simulink library "vlbi_lib"  (Simulink 7.3)
settings: Solver=ode45  SolverMode=SingleTasking  StartTime=0.0  StopTime=10.0  RelTol=1e-3
libraries: xbsIndex_r4 x437, xbsReplacements_r4 x26, simulink x3, xps_library x2
(part 2 of 2)

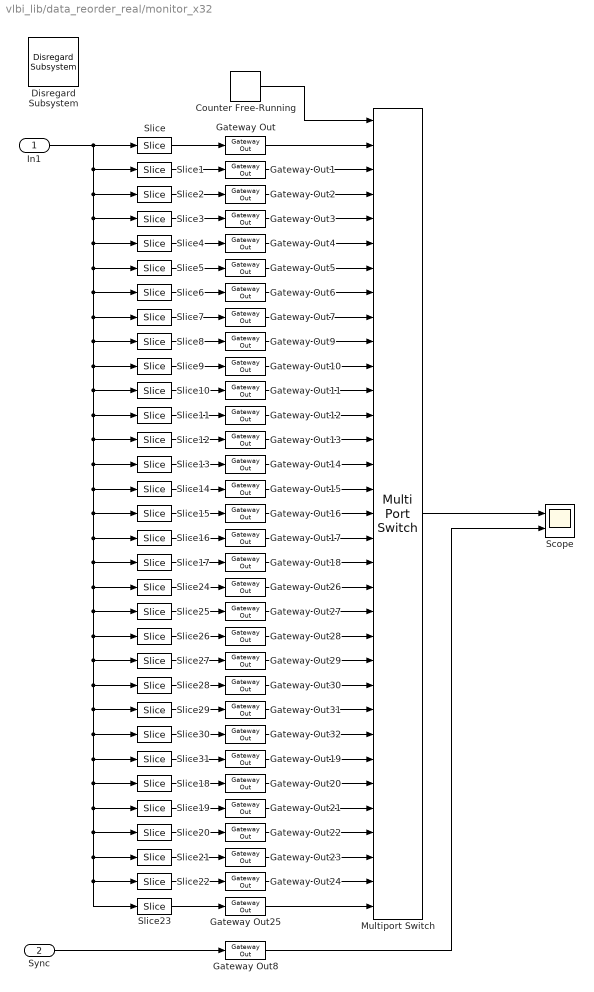
== system vlbi_lib/data_reorder_real/monitor_x32 ==
  In1 : Inport  OutDataType=sfix(16)  OutScaling=2^0
  Sync : Inport  Port=2  OutDataType=sfix(16)  OutScaling=2^0
  Counter Free-Running : simulink/Sources/Counter Free-Running  SystemSampleTime=-1  NumBits=5  tsamp=1/32
  Disregard Subsystem : xbsIndex_r4/Disregard Subsystem  Tag=discardX  block_type=disregard
      settings: block_version=11.3
  Gateway Out{,1..32} (33 alike) : xbsIndex_r4/Gateway Out  hdl_port=off  timing_constraint=None  locs_specified=off  LOCs={}  block_type=gatewayout
      settings: infoedit="Gateway out block.  Converts Xilinx fixed point inputs into ouputs of type Simulink integer, double, or fixed point.<br><br>Hardware notes:  In hardware these blocks become top level output ports or are discarded, depending on how they are configured."  xl_area=[0, 0, 0, 0, 0, 0, 0]  block_version=11.3
  Multiport Switch : MultiPortSwitch  Inputs=32  zeroidx=on  SampleTime=1/32
  Scope : Scope  NumInputPorts=2
      settings: YMin=-5~-5  YMax=5~5
  Slice : xbsIndex_r4/Slice  nbits=sample_width  boolean_output=off  mode=Lower Bit Location + Width  bit1=sample_width*0  base1=MSB of Input  bit0=sample_width*7  base0=LSB of Input  dbl_ovrd=off  block_type=slice
      settings: block_version=11.3
  Slice1 : xbsIndex_r4/Slice  nbits=sample_width  boolean_output=off  mode=Lower Bit Location + Width  bit1=-2*sample_width  base1=MSB of Input  bit0=sample_width*6  base0=LSB of Input  dbl_ovrd=off  block_type=slice
      settings: block_version=11.3
  Slice10 : xbsIndex_r4/Slice  nbits=sample_width  boolean_output=off  mode=Lower Bit Location + Width  bit1=sample_width*21  base1=MSB of Input  bit0=sample_width*21  base0=LSB of Input  dbl_ovrd=off  block_type=slice
      settings: block_version=11.3
  Slice11 : xbsIndex_r4/Slice  nbits=sample_width  boolean_output=off  mode=Lower Bit Location + Width  bit1=-22*sample_width  base1=MSB of Input  bit0=sample_width*20  base0=LSB of Input  dbl_ovrd=off  block_type=slice
      settings: block_version=11.3
  Slice12 : xbsIndex_r4/Slice  nbits=sample_width  boolean_output=off  mode=Lower Bit Location + Width  bit1=-24*sample_width  base1=MSB of Input  bit0=sample_width*31  base0=LSB of Input  dbl_ovrd=off  block_type=slice
      settings: block_version=11.3
  Slice13 : xbsIndex_r4/Slice  nbits=sample_width  boolean_output=off  mode=Lower Bit Location + Width  bit1=-26*sample_width  base1=MSB of Input  bit0=sample_width*30  base0=LSB of Input  dbl_ovrd=off  block_type=slice
      settings: block_version=11.3
  Slice14 : xbsIndex_r4/Slice  nbits=sample_width  boolean_output=off  mode=Lower Bit Location + Width  bit1=-28*sample_width  base1=MSB of Input  bit0=sample_width*29  base0=LSB of Input  dbl_ovrd=off  block_type=slice
      settings: block_version=11.3
  Slice15 : xbsIndex_r4/Slice  nbits=sample_width  boolean_output=off  mode=Lower Bit Location + Width  bit1=-30*sample_width  base1=MSB of Input  bit0=sample_width*28  base0=LSB of Input  dbl_ovrd=off  block_type=slice
      settings: block_version=11.3
  Slice16 : xbsIndex_r4/Slice  nbits=sample_width  boolean_output=off  mode=Lower Bit Location + Width  bit1=-1*sample_width  base1=MSB of Input  bit0=sample_width*3  base0=LSB of Input  dbl_ovrd=off  block_type=slice
      settings: block_version=11.3
  Slice17 : xbsIndex_r4/Slice  nbits=sample_width  boolean_output=off  mode=Lower Bit Location + Width  bit1=-3*sample_width  base1=MSB of Input  bit0=sample_width*2  base0=LSB of Input  dbl_ovrd=off  block_type=slice
      settings: block_version=11.3
  Slice18 : xbsIndex_r4/Slice  nbits=sample_width  boolean_output=off  mode=Lower Bit Location + Width  bit1=-21*sample_width  base1=MSB of Input  bit0=sample_width*17  base0=LSB of Input  dbl_ovrd=off  block_type=slice
      settings: block_version=11.3
  Slice19 : xbsIndex_r4/Slice  nbits=sample_width  boolean_output=off  mode=Lower Bit Location + Width  bit1=-23*sample_width  base1=MSB of Input  bit0=sample_width*16  base0=LSB of Input  dbl_ovrd=off  block_type=slice
      settings: block_version=11.3
  Slice2 : xbsIndex_r4/Slice  nbits=sample_width  boolean_output=off  mode=Lower Bit Location + Width  bit1=-4*sample_width  base1=MSB of Input  bit0=sample_width*5  base0=LSB of Input  dbl_ovrd=off  block_type=slice
      settings: block_version=11.3
  Slice20 : xbsIndex_r4/Slice  nbits=sample_width  boolean_output=off  mode=Lower Bit Location + Width  bit1=-25*sample_width  base1=MSB of Input  bit0=sample_width*27  base0=LSB of Input  dbl_ovrd=off  block_type=slice
      settings: block_version=11.3
  Slice21 : xbsIndex_r4/Slice  nbits=sample_width  boolean_output=off  mode=Lower Bit Location + Width  bit1=-27*sample_width  base1=MSB of Input  bit0=sample_width*26  base0=LSB of Input  dbl_ovrd=off  block_type=slice
      settings: block_version=11.3
  Slice22 : xbsIndex_r4/Slice  nbits=sample_width  boolean_output=off  mode=Lower Bit Location + Width  bit1=-29*sample_width  base1=MSB of Input  bit0=sample_width*25  base0=LSB of Input  dbl_ovrd=off  block_type=slice
      settings: block_version=11.3
  Slice23 : xbsIndex_r4/Slice  nbits=sample_width  boolean_output=off  mode=Lower Bit Location + Width  bit1=-31*sample_width  base1=MSB of Input  bit0=sample_width*24  base0=LSB of Input  dbl_ovrd=off  block_type=slice
      settings: block_version=11.3
  Slice24 : xbsIndex_r4/Slice  nbits=sample_width  boolean_output=off  mode=Lower Bit Location + Width  bit1=-5*sample_width  base1=MSB of Input  bit0=sample_width*1  base0=LSB of Input  dbl_ovrd=off  block_type=slice
      settings: block_version=11.3
  Slice25 : xbsIndex_r4/Slice  nbits=sample_width  boolean_output=off  mode=Lower Bit Location + Width  bit1=-7*sample_width  base1=MSB of Input  bit0=sample_width*0  base0=LSB of Input  dbl_ovrd=off  block_type=slice
      settings: block_version=11.3
  Slice26 : xbsIndex_r4/Slice  nbits=sample_width  boolean_output=off  mode=Lower Bit Location + Width  bit1=-9*sample_width  base1=MSB of Input  bit0=sample_width*11  base0=LSB of Input  dbl_ovrd=off  block_type=slice
      settings: block_version=11.3
  Slice27 : xbsIndex_r4/Slice  nbits=sample_width  boolean_output=off  mode=Lower Bit Location + Width  bit1=-11*sample_width  base1=MSB of Input  bit0=sample_width*10  base0=LSB of Input  dbl_ovrd=off  block_type=slice
      settings: block_version=11.3
  Slice28 : xbsIndex_r4/Slice  nbits=sample_width  boolean_output=off  mode=Lower Bit Location + Width  bit1=-13*sample_width  base1=MSB of Input  bit0=sample_width*9  base0=LSB of Input  dbl_ovrd=off  block_type=slice
      settings: block_version=11.3
  Slice29 : xbsIndex_r4/Slice  nbits=sample_width  boolean_output=off  mode=Lower Bit Location + Width  bit1=-15*sample_width  base1=MSB of Input  bit0=sample_width*8  base0=LSB of Input  dbl_ovrd=off  block_type=slice
      settings: block_version=11.3
  Slice3 : xbsIndex_r4/Slice  nbits=sample_width  boolean_output=off  mode=Lower Bit Location + Width  bit1=-6*sample_width  base1=MSB of Input  bit0=sample_width*4  base0=LSB of Input  dbl_ovrd=off  block_type=slice
      settings: block_version=11.3
  Slice30 : xbsIndex_r4/Slice  nbits=sample_width  boolean_output=off  mode=Lower Bit Location + Width  bit1=-17*sample_width  base1=MSB of Input  bit0=sample_width*19  base0=LSB of Input  dbl_ovrd=off  block_type=slice
      settings: block_version=11.3
  Slice31 : xbsIndex_r4/Slice  nbits=sample_width  boolean_output=off  mode=Lower Bit Location + Width  bit1=sample_width*18  base1=MSB of Input  bit0=sample_width*18  base0=LSB of Input  dbl_ovrd=off  block_type=slice
      settings: block_version=11.3
  Slice4 : xbsIndex_r4/Slice  nbits=sample_width  boolean_output=off  mode=Lower Bit Location + Width  bit1=-8*sample_width  base1=MSB of Input  bit0=sample_width*15  base0=LSB of Input  dbl_ovrd=off  block_type=slice
      settings: block_version=11.3
  Slice5 : xbsIndex_r4/Slice  nbits=sample_width  boolean_output=off  mode=Lower Bit Location + Width  bit1=-10*sample_width  base1=MSB of Input  bit0=sample_width*14  base0=LSB of Input  dbl_ovrd=off  block_type=slice
      settings: block_version=11.3
  Slice6 : xbsIndex_r4/Slice  nbits=sample_width  boolean_output=off  mode=Lower Bit Location + Width  bit1=-12*sample_width  base1=MSB of Input  bit0=sample_width*13  base0=LSB of Input  dbl_ovrd=off  block_type=slice
      settings: block_version=11.3
  Slice7 : xbsIndex_r4/Slice  nbits=sample_width  boolean_output=off  mode=Lower Bit Location + Width  bit1=-14*sample_width  base1=MSB of Input  bit0=sample_width*12  base0=LSB of Input  dbl_ovrd=off  block_type=slice
      settings: block_version=11.3
  Slice8 : xbsIndex_r4/Slice  nbits=sample_width  boolean_output=off  mode=Lower Bit Location + Width  bit1=-16*sample_width  base1=MSB of Input  bit0=sample_width*23  base0=LSB of Input  dbl_ovrd=off  block_type=slice
      settings: block_version=11.3
  Slice9 : xbsIndex_r4/Slice  nbits=sample_width  boolean_output=off  mode=Lower Bit Location + Width  bit1=-18*sample_width  base1=MSB of Input  bit0=sample_width*22  base0=LSB of Input  dbl_ovrd=off  block_type=slice
      settings: block_version=11.3
  wires:
  Gateway Out8/1 -> Scope/2
  Sync/1 -> Gateway Out8/1
  Multiport Switch/1 -> Scope/1
  Counter Free-Running/1 -> Multiport Switch/1
  Slice7/1 -> Gateway Out7/1
  Slice6/1 -> Gateway Out6/1
  Slice5/1 -> Gateway Out5/1
  Slice4/1 -> Gateway Out4/1
  Slice3/1 -> Gateway Out3/1
  Slice2/1 -> Gateway Out2/1
  Slice1/1 -> Gateway Out1/1
  Slice/1 -> Gateway Out/1
  In1/1 -> Slice6/1, Slice7/1, Slice14/1, Slice15/1, Slice16/1, Slice17/1, Slice24/1, Slice25/1, Slice26/1, Slice27/1, Slice30/1, Slice31/1, Slice18/1, Slice19/1, Slice20/1, Slice21/1, Slice22/1, Slice23/1, Slice29/1, Slice28/1, Slice13/1, Slice12/1, Slice11/1, Slice10/1, Slice9/1, Slice8/1, Slice5/1, Slice4/1, Slice3/1, Slice2/1, Slice1/1, Slice/1
  Slice15/1 -> Gateway Out16/1
  Slice14/1 -> Gateway Out15/1
  Slice13/1 -> Gateway Out14/1
  Slice12/1 -> Gateway Out13/1
  Slice11/1 -> Gateway Out12/1
  Slice10/1 -> Gateway Out11/1
  Slice9/1 -> Gateway Out10/1
  Slice8/1 -> Gateway Out9/1
  Slice29/1 -> Gateway Out31/1
  Slice28/1 -> Gateway Out30/1
  Slice27/1 -> Gateway Out29/1
  Slice26/1 -> Gateway Out28/1
  Slice25/1 -> Gateway Out27/1
  Slice24/1 -> Gateway Out26/1
  Slice17/1 -> Gateway Out18/1
  Slice16/1 -> Gateway Out17/1
  Slice23/1 -> Gateway Out25/1
  Slice22/1 -> Gateway Out24/1
  Slice21/1 -> Gateway Out23/1
  Slice20/1 -> Gateway Out22/1
  Slice19/1 -> Gateway Out21/1
  Slice18/1 -> Gateway Out20/1
  Slice31/1 -> Gateway Out19/1
  Slice30/1 -> Gateway Out32/1
  Gateway Out/1 -> Multiport Switch/2
  Gateway Out1/1 -> Multiport Switch/3
  Gateway Out2/1 -> Multiport Switch/4
  Gateway Out3/1 -> Multiport Switch/5
  Gateway Out4/1 -> Multiport Switch/6
  Gateway Out5/1 -> Multiport Switch/7
  Gateway Out6/1 -> Multiport Switch/8
  Gateway Out7/1 -> Multiport Switch/9
  Gateway Out9/1 -> Multiport Switch/10
  Gateway Out10/1 -> Multiport Switch/11
  Gateway Out11/1 -> Multiport Switch/12
  Gateway Out12/1 -> Multiport Switch/13
  Gateway Out13/1 -> Multiport Switch/14
  Gateway Out14/1 -> Multiport Switch/15
  Gateway Out15/1 -> Multiport Switch/16
  Gateway Out16/1 -> Multiport Switch/17
  Gateway Out17/1 -> Multiport Switch/18
  Gateway Out18/1 -> Multiport Switch/19
  Gateway Out26/1 -> Multiport Switch/20
  Gateway Out27/1 -> Multiport Switch/21
  Gateway Out28/1 -> Multiport Switch/22
  Gateway Out29/1 -> Multiport Switch/23
  Gateway Out30/1 -> Multiport Switch/24
  Gateway Out31/1 -> Multiport Switch/25
  Gateway Out32/1 -> Multiport Switch/26
  Gateway Out19/1 -> Multiport Switch/27
  Gateway Out20/1 -> Multiport Switch/28
  Gateway Out21/1 -> Multiport Switch/29
  Gateway Out22/1 -> Multiport Switch/30
  Gateway Out23/1 -> Multiport Switch/31
  Gateway Out24/1 -> Multiport Switch/32
  Gateway Out25/1 -> Multiport Switch/33

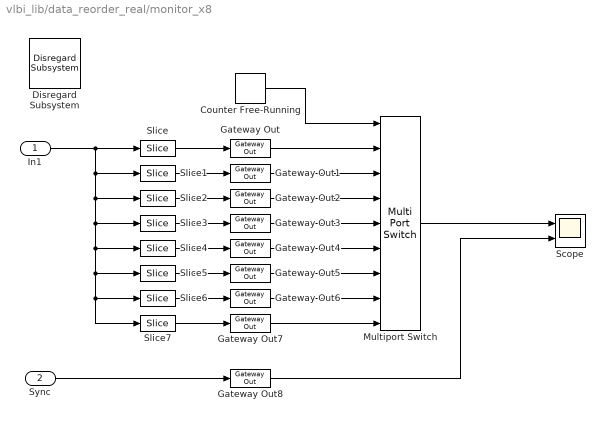
== system vlbi_lib/data_reorder_real/monitor_x8 ==
  In1 : Inport  OutDataType=sfix(16)  OutScaling=2^0
  Sync : Inport  Port=2  OutDataType=sfix(16)  OutScaling=2^0
  Counter Free-Running : simulink/Sources/Counter Free-Running  SystemSampleTime=-1  NumBits=3  tsamp=1/8
  Disregard Subsystem : xbsIndex_r4/Disregard Subsystem  Tag=discardX  block_type=disregard
      settings: block_version=11.3
  Gateway Out{,1..8} (9 alike) : xbsIndex_r4/Gateway Out  hdl_port=off  timing_constraint=None  locs_specified=off  LOCs={}  block_type=gatewayout
      settings: infoedit="Gateway out block.  Converts Xilinx fixed point inputs into ouputs of type Simulink integer, double, or fixed point.<br><br>Hardware notes:  In hardware these blocks become top level output ports or are discarded, depending on how they are configured."  xl_area=[0, 0, 0, 0, 0, 0, 0]  block_version=11.3
  Multiport Switch : MultiPortSwitch  Inputs=8  zeroidx=on  SampleTime=1/8
  Scope : Scope  NumInputPorts=2
      settings: YMin=-5~-5  YMax=5~5
  Slice : xbsIndex_r4/Slice  nbits=sample_width  boolean_output=off  mode=Upper Bit Location + Width  bit1=0  base1=MSB of Input  bit0=0  base0=LSB of Input  dbl_ovrd=off  block_type=slice
      settings: block_version=11.3
  Slice1 : xbsIndex_r4/Slice  nbits=sample_width  boolean_output=off  mode=Upper Bit Location + Width  bit1=-1*sample_width  base1=MSB of Input  bit0=0  base0=LSB of Input  dbl_ovrd=off  block_type=slice
      settings: block_version=11.3
  Slice2 : xbsIndex_r4/Slice  nbits=sample_width  boolean_output=off  mode=Upper Bit Location + Width  bit1=-2*sample_width  base1=MSB of Input  bit0=0  base0=LSB of Input  dbl_ovrd=off  block_type=slice
      settings: block_version=11.3
  Slice3 : xbsIndex_r4/Slice  nbits=sample_width  boolean_output=off  mode=Upper Bit Location + Width  bit1=-3*sample_width  base1=MSB of Input  bit0=0  base0=LSB of Input  dbl_ovrd=off  block_type=slice
      settings: block_version=11.3
  Slice4 : xbsIndex_r4/Slice  nbits=sample_width  boolean_output=off  mode=Upper Bit Location + Width  bit1=-4*sample_width  base1=MSB of Input  bit0=0  base0=LSB of Input  dbl_ovrd=off  block_type=slice
      settings: block_version=11.3
  Slice5 : xbsIndex_r4/Slice  nbits=sample_width  boolean_output=off  mode=Upper Bit Location + Width  bit1=-5*sample_width  base1=MSB of Input  bit0=0  base0=LSB of Input  dbl_ovrd=off  block_type=slice
      settings: block_version=11.3
  Slice6 : xbsIndex_r4/Slice  nbits=sample_width  boolean_output=off  mode=Upper Bit Location + Width  bit1=-6*sample_width  base1=MSB of Input  bit0=0  base0=LSB of Input  dbl_ovrd=off  block_type=slice
      settings: block_version=11.3
  Slice7 : xbsIndex_r4/Slice  nbits=sample_width  boolean_output=off  mode=Upper Bit Location + Width  bit1=-7*sample_width  base1=MSB of Input  bit0=0  base0=LSB of Input  dbl_ovrd=off  block_type=slice
      settings: block_version=11.3
  wires:
  In1/1 -> Slice/1, Slice1/1, Slice2/1, Slice3/1, Slice4/1, Slice5/1, Slice6/1, Slice7/1
  Slice/1 -> Gateway Out/1
  Slice1/1 -> Gateway Out1/1
  Slice2/1 -> Gateway Out2/1
  Slice3/1 -> Gateway Out3/1
  Slice4/1 -> Gateway Out4/1
  Slice5/1 -> Gateway Out5/1
  Slice6/1 -> Gateway Out6/1
  Slice7/1 -> Gateway Out7/1
  Counter Free-Running/1 -> Multiport Switch/1
  Gateway Out/1 -> Multiport Switch/2
  Gateway Out1/1 -> Multiport Switch/3
  Gateway Out2/1 -> Multiport Switch/4
  Gateway Out3/1 -> Multiport Switch/5
  Gateway Out4/1 -> Multiport Switch/6
  Gateway Out5/1 -> Multiport Switch/7
  Gateway Out6/1 -> Multiport Switch/8
  Gateway Out7/1 -> Multiport Switch/9
  Multiport Switch/1 -> Scope/1
  Sync/1 -> Gateway Out8/1
  Gateway Out8/1 -> Scope/2

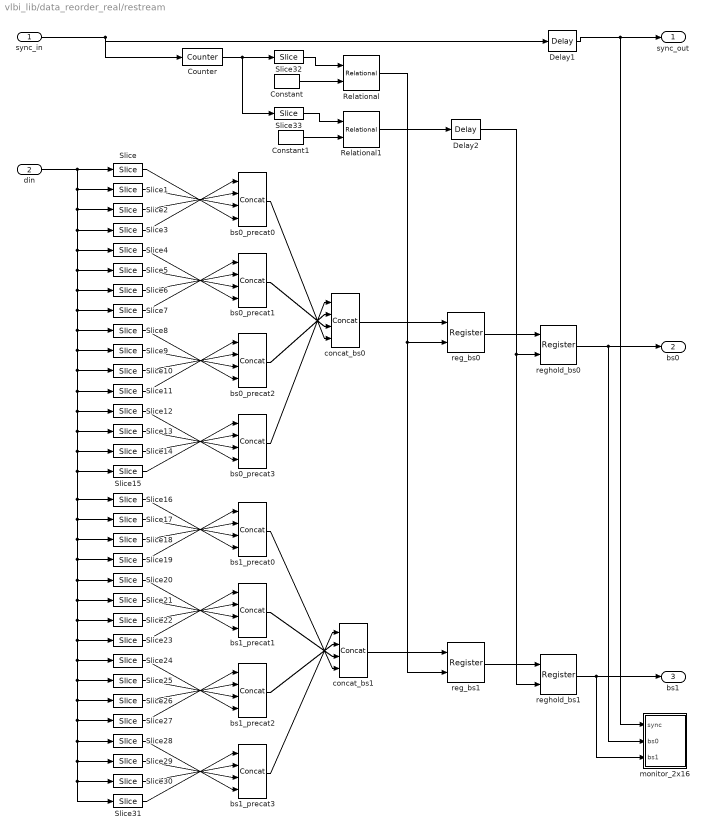
== system vlbi_lib/data_reorder_real/restream ==
  sync_in : Inport  OutDataType=sfix(16)  OutScaling=2^0
  din : Inport  Port=2  OutDataType=sfix(16)  OutScaling=2^0
  Constant : xbsIndex_r4/Constant  arith_type=Unsigned  const=0  n_bits=8-log2(clock_rate)  bin_pt=0  explicit_period=on  period=1  equ=P=C  opselect=C  inp2=PCIN>>17  opr=+  inp1=P  carry=CIN  dbl_ovrd=off  block_type=constant
      settings: block_version=11.3
  Constant1 : xbsIndex_r4/Constant  arith_type=Unsigned  const=0  n_bits=8-log2(clock_rate)  bin_pt=0  explicit_period=on  period=1  equ=P=C  opselect=C  inp2=PCIN>>17  opr=+  inp1=P  carry=CIN  dbl_ovrd=off  block_type=constant
      settings: block_version=11.3
  Counter : xbsIndex_r4/Counter  cnt_type=Free Running  cnt_to=Inf  operation=Up  start_count=0  cnt_by_val=1  arith_type=Unsigned  n_bits=9-log2(clock_rate)  bin_pt=0  load_pin=off  rst=on  en=off  explicit_period=off  period=1  dbl_ovrd=off  use_behavioral_HDL=off  implementation=Fabric  use_rpm=on  block_type=counter
      settings: xl_area=[0, 0, 0, 0, 0, 0, 0]  block_version=11.3
  Delay1 : xbsIndex_r4/Delay  en=off  latency=2  dbl_ovrd=off  reg_retiming=off  block_type=delay
      settings: xl_area=[0, 0, 0, 0, 0, 0, 0]  block_version=11.3
  Delay2 : xbsIndex_r4/Delay  en=off  latency=1  dbl_ovrd=off  reg_retiming=off  block_type=delay
      settings: xl_area=[0, 0, 0, 0, 0, 0, 0]  block_version=11.3
  Relational : xbsIndex_r4/Relational  mode=a=b  en=off  latency=0  dbl_ovrd=off  block_type=relational
      settings: xl_area=[0, 0, 0, 0, 0, 0, 0]  block_version=11.3
  Relational1 : xbsIndex_r4/Relational  mode=a=b  en=off  latency=0  dbl_ovrd=off  block_type=relational
      settings: xl_area=[0, 0, 0, 0, 0, 0, 0]  block_version=11.3
  Slice : xbsIndex_r4/Slice  nbits=sample_width  boolean_output=off  mode=Lower Bit Location + Width  bit1=sample_width*0  base1=MSB of Input  bit0=sample_width*7  base0=LSB of Input  dbl_ovrd=off  block_type=slice
      settings: block_version=11.3
  Slice1 : xbsIndex_r4/Slice  nbits=sample_width  boolean_output=off  mode=Lower Bit Location + Width  bit1=-2*sample_width  base1=MSB of Input  bit0=sample_width*6  base0=LSB of Input  dbl_ovrd=off  block_type=slice
      settings: block_version=11.3
  Slice10 : xbsIndex_r4/Slice  nbits=sample_width  boolean_output=off  mode=Lower Bit Location + Width  bit1=sample_width*21  base1=MSB of Input  bit0=sample_width*21  base0=LSB of Input  dbl_ovrd=off  block_type=slice
      settings: block_version=11.3
  Slice11 : xbsIndex_r4/Slice  nbits=sample_width  boolean_output=off  mode=Lower Bit Location + Width  bit1=-22*sample_width  base1=MSB of Input  bit0=sample_width*20  base0=LSB of Input  dbl_ovrd=off  block_type=slice
      settings: block_version=11.3
  Slice12 : xbsIndex_r4/Slice  nbits=sample_width  boolean_output=off  mode=Lower Bit Location + Width  bit1=-24*sample_width  base1=MSB of Input  bit0=sample_width*31  base0=LSB of Input  dbl_ovrd=off  block_type=slice
      settings: block_version=11.3
  Slice13 : xbsIndex_r4/Slice  nbits=sample_width  boolean_output=off  mode=Lower Bit Location + Width  bit1=-26*sample_width  base1=MSB of Input  bit0=sample_width*30  base0=LSB of Input  dbl_ovrd=off  block_type=slice
      settings: block_version=11.3
  Slice14 : xbsIndex_r4/Slice  nbits=sample_width  boolean_output=off  mode=Lower Bit Location + Width  bit1=-28*sample_width  base1=MSB of Input  bit0=sample_width*29  base0=LSB of Input  dbl_ovrd=off  block_type=slice
      settings: block_version=11.3
  Slice15 : xbsIndex_r4/Slice  nbits=sample_width  boolean_output=off  mode=Lower Bit Location + Width  bit1=-30*sample_width  base1=MSB of Input  bit0=sample_width*28  base0=LSB of Input  dbl_ovrd=off  block_type=slice
      settings: block_version=11.3
  Slice16 : xbsIndex_r4/Slice  nbits=sample_width  boolean_output=off  mode=Lower Bit Location + Width  bit1=-1*sample_width  base1=MSB of Input  bit0=sample_width*3  base0=LSB of Input  dbl_ovrd=off  block_type=slice
      settings: block_version=11.3
  Slice17 : xbsIndex_r4/Slice  nbits=sample_width  boolean_output=off  mode=Lower Bit Location + Width  bit1=-3*sample_width  base1=MSB of Input  bit0=sample_width*2  base0=LSB of Input  dbl_ovrd=off  block_type=slice
      settings: block_version=11.3
  Slice18 : xbsIndex_r4/Slice  nbits=sample_width  boolean_output=off  mode=Lower Bit Location + Width  bit1=-5*sample_width  base1=MSB of Input  bit0=sample_width*1  base0=LSB of Input  dbl_ovrd=off  block_type=slice
      settings: block_version=11.3
  Slice19 : xbsIndex_r4/Slice  nbits=sample_width  boolean_output=off  mode=Lower Bit Location + Width  bit1=-7*sample_width  base1=MSB of Input  bit0=sample_width*0  base0=LSB of Input  dbl_ovrd=off  block_type=slice
      settings: block_version=11.3
  Slice2 : xbsIndex_r4/Slice  nbits=sample_width  boolean_output=off  mode=Lower Bit Location + Width  bit1=-4*sample_width  base1=MSB of Input  bit0=sample_width*5  base0=LSB of Input  dbl_ovrd=off  block_type=slice
      settings: block_version=11.3
  Slice20 : xbsIndex_r4/Slice  nbits=sample_width  boolean_output=off  mode=Lower Bit Location + Width  bit1=-9*sample_width  base1=MSB of Input  bit0=sample_width*11  base0=LSB of Input  dbl_ovrd=off  block_type=slice
      settings: block_version=11.3
  Slice21 : xbsIndex_r4/Slice  nbits=sample_width  boolean_output=off  mode=Lower Bit Location + Width  bit1=-11*sample_width  base1=MSB of Input  bit0=sample_width*10  base0=LSB of Input  dbl_ovrd=off  block_type=slice
      settings: block_version=11.3
  Slice22 : xbsIndex_r4/Slice  nbits=sample_width  boolean_output=off  mode=Lower Bit Location + Width  bit1=-13*sample_width  base1=MSB of Input  bit0=sample_width*9  base0=LSB of Input  dbl_ovrd=off  block_type=slice
      settings: block_version=11.3
  Slice23 : xbsIndex_r4/Slice  nbits=sample_width  boolean_output=off  mode=Lower Bit Location + Width  bit1=-15*sample_width  base1=MSB of Input  bit0=sample_width*8  base0=LSB of Input  dbl_ovrd=off  block_type=slice
      settings: block_version=11.3
  Slice24 : xbsIndex_r4/Slice  nbits=sample_width  boolean_output=off  mode=Lower Bit Location + Width  bit1=-17*sample_width  base1=MSB of Input  bit0=sample_width*19  base0=LSB of Input  dbl_ovrd=off  block_type=slice
      settings: block_version=11.3
  Slice25 : xbsIndex_r4/Slice  nbits=sample_width  boolean_output=off  mode=Lower Bit Location + Width  bit1=sample_width*18  base1=MSB of Input  bit0=sample_width*18  base0=LSB of Input  dbl_ovrd=off  block_type=slice
      settings: block_version=11.3
  Slice26 : xbsIndex_r4/Slice  nbits=sample_width  boolean_output=off  mode=Lower Bit Location + Width  bit1=-21*sample_width  base1=MSB of Input  bit0=sample_width*17  base0=LSB of Input  dbl_ovrd=off  block_type=slice
      settings: block_version=11.3
  Slice27 : xbsIndex_r4/Slice  nbits=sample_width  boolean_output=off  mode=Lower Bit Location + Width  bit1=-23*sample_width  base1=MSB of Input  bit0=sample_width*16  base0=LSB of Input  dbl_ovrd=off  block_type=slice
      settings: block_version=11.3
  Slice28 : xbsIndex_r4/Slice  nbits=sample_width  boolean_output=off  mode=Lower Bit Location + Width  bit1=-25*sample_width  base1=MSB of Input  bit0=sample_width*27  base0=LSB of Input  dbl_ovrd=off  block_type=slice
      settings: block_version=11.3
  Slice29 : xbsIndex_r4/Slice  nbits=sample_width  boolean_output=off  mode=Lower Bit Location + Width  bit1=-27*sample_width  base1=MSB of Input  bit0=sample_width*26  base0=LSB of Input  dbl_ovrd=off  block_type=slice
      settings: block_version=11.3
  Slice3 : xbsIndex_r4/Slice  nbits=sample_width  boolean_output=off  mode=Lower Bit Location + Width  bit1=-6*sample_width  base1=MSB of Input  bit0=sample_width*4  base0=LSB of Input  dbl_ovrd=off  block_type=slice
      settings: block_version=11.3
  Slice30 : xbsIndex_r4/Slice  nbits=sample_width  boolean_output=off  mode=Lower Bit Location + Width  bit1=-29*sample_width  base1=MSB of Input  bit0=sample_width*25  base0=LSB of Input  dbl_ovrd=off  block_type=slice
      settings: block_version=11.3
  Slice31 : xbsIndex_r4/Slice  nbits=sample_width  boolean_output=off  mode=Lower Bit Location + Width  bit1=-31*sample_width  base1=MSB of Input  bit0=sample_width*24  base0=LSB of Input  dbl_ovrd=off  block_type=slice
      settings: block_version=11.3
  Slice32 : xbsIndex_r4/Slice  nbits=8-log2(clock_rate)  boolean_output=off  mode=Upper Bit Location + Width  bit1=0  base1=MSB of Input  bit0=sample_width*7  base0=LSB of Input  dbl_ovrd=off  block_type=slice
      settings: block_version=11.3
  Slice33 : xbsIndex_r4/Slice  nbits=8-log2(clock_rate)  boolean_output=off  mode=Lower Bit Location + Width  bit1=0  base1=MSB of Input  bit0=0  base0=LSB of Input  dbl_ovrd=off  block_type=slice
      settings: block_version=11.3
  Slice4 : xbsIndex_r4/Slice  nbits=sample_width  boolean_output=off  mode=Lower Bit Location + Width  bit1=-8*sample_width  base1=MSB of Input  bit0=sample_width*15  base0=LSB of Input  dbl_ovrd=off  block_type=slice
      settings: block_version=11.3
  Slice5 : xbsIndex_r4/Slice  nbits=sample_width  boolean_output=off  mode=Lower Bit Location + Width  bit1=-10*sample_width  base1=MSB of Input  bit0=sample_width*14  base0=LSB of Input  dbl_ovrd=off  block_type=slice
      settings: block_version=11.3
  Slice6 : xbsIndex_r4/Slice  nbits=sample_width  boolean_output=off  mode=Lower Bit Location + Width  bit1=-12*sample_width  base1=MSB of Input  bit0=sample_width*13  base0=LSB of Input  dbl_ovrd=off  block_type=slice
      settings: block_version=11.3
  Slice7 : xbsIndex_r4/Slice  nbits=sample_width  boolean_output=off  mode=Lower Bit Location + Width  bit1=-14*sample_width  base1=MSB of Input  bit0=sample_width*12  base0=LSB of Input  dbl_ovrd=off  block_type=slice
      settings: block_version=11.3
  Slice8 : xbsIndex_r4/Slice  nbits=sample_width  boolean_output=off  mode=Lower Bit Location + Width  bit1=-16*sample_width  base1=MSB of Input  bit0=sample_width*23  base0=LSB of Input  dbl_ovrd=off  block_type=slice
      settings: block_version=11.3
  Slice9 : xbsIndex_r4/Slice  nbits=sample_width  boolean_output=off  mode=Lower Bit Location + Width  bit1=-18*sample_width  base1=MSB of Input  bit0=sample_width*22  base0=LSB of Input  dbl_ovrd=off  block_type=slice
      settings: block_version=11.3
  bs0_precat{0..3} (4 alike) : xbsIndex_r4/Concat  num_inputs=4  dbl_ovrd=off  block_type=concat
      settings: block_version=11.3
  bs1_precat{0..3} (4 alike) : xbsIndex_r4/Concat  num_inputs=4  dbl_ovrd=off  block_type=concat
      settings: block_version=11.3
  concat_bs0 : xbsIndex_r4/Concat  num_inputs=4  dbl_ovrd=off  block_type=concat
      settings: block_version=11.3
  concat_bs1 : xbsIndex_r4/Concat  num_inputs=4  dbl_ovrd=off  block_type=concat
      settings: block_version=11.3
  monitor_2x16 : Subsystem
  reg_bs0 : xbsIndex_r4/Register  init=0  rst=off  en=on  dbl_ovrd=off  block_type=register
      settings: xl_area=[0, 0, 0, 0, 0, 0, 0]  block_version=11.3
  reg_bs1 : xbsIndex_r4/Register  init=0  rst=off  en=on  dbl_ovrd=off  block_type=register
      settings: xl_area=[0, 0, 0, 0, 0, 0, 0]  block_version=11.3
  reghold_bs0 : xbsIndex_r4/Register  init=0  rst=off  en=on  dbl_ovrd=off  block_type=register
      settings: xl_area=[0, 0, 0, 0, 0, 0, 0]  block_version=11.3
  reghold_bs1 : xbsIndex_r4/Register  init=0  rst=off  en=on  dbl_ovrd=off  block_type=register
      settings: xl_area=[0, 0, 0, 0, 0, 0, 0]  block_version=11.3
  sync_out : Outport  OutDataType=sfix(16)  OutScaling=2^0
  bs0 : Outport  Port=2  OutDataType=sfix(16)  OutScaling=2^0
  bs1 : Outport  Port=3  OutDataType=sfix(16)  OutScaling=2^0
  wires:
  bs1_precat3/1 -> concat_bs1/1
  bs1_precat2/1 -> concat_bs1/2
  bs1_precat1/1 -> concat_bs1/3
  bs1_precat0/1 -> concat_bs1/4
  bs0_precat3/1 -> concat_bs0/1
  bs0_precat2/1 -> concat_bs0/2
  bs0_precat1/1 -> concat_bs0/3
  bs0_precat0/1 -> concat_bs0/4
  concat_bs1/1 -> reg_bs1/1
  concat_bs0/1 -> reg_bs0/1
  Slice31/1 -> bs1_precat3/1
  Slice30/1 -> bs1_precat3/2
  Slice29/1 -> bs1_precat3/3
  Slice28/1 -> bs1_precat3/4
  Slice27/1 -> bs1_precat2/1
  Slice26/1 -> bs1_precat2/2
  Slice25/1 -> bs1_precat2/3
  Slice24/1 -> bs1_precat2/4
  Slice23/1 -> bs1_precat1/1
  Slice22/1 -> bs1_precat1/2
  Slice21/1 -> bs1_precat1/3
  Slice20/1 -> bs1_precat1/4
  Slice19/1 -> bs1_precat0/1
  Slice18/1 -> bs1_precat0/2
  Slice17/1 -> bs1_precat0/3
  Slice16/1 -> bs1_precat0/4
  Slice15/1 -> bs0_precat3/1
  Slice14/1 -> bs0_precat3/2
  Slice13/1 -> bs0_precat3/3
  Slice12/1 -> bs0_precat3/4
  Slice11/1 -> bs0_precat2/1
  Slice10/1 -> bs0_precat2/2
  Slice9/1 -> bs0_precat2/3
  Slice8/1 -> bs0_precat2/4
  Slice7/1 -> bs0_precat1/1
  Slice6/1 -> bs0_precat1/2
  Slice5/1 -> bs0_precat1/3
  Slice4/1 -> bs0_precat1/4
  Slice3/1 -> bs0_precat0/1
  Slice2/1 -> bs0_precat0/2
  Slice1/1 -> bs0_precat0/3
  Slice/1 -> bs0_precat0/4
  din/1 -> Slice/1, Slice1/1, Slice2/1, Slice3/1, Slice4/1, Slice5/1, Slice8/1, Slice9/1, Slice10/1, Slice11/1, Slice12/1, Slice13/1, Slice22/1, Slice23/1, Slice31/1, Slice30/1, Slice29/1, Slice28/1, Slice27/1, Slice26/1, Slice25/1, Slice24/1, Slice21/1, Slice20/1, Slice19/1, Slice18/1, Slice17/1, Slice16/1, Slice15/1, Slice14/1, Slice7/1, Slice6/1
  sync_in/1 -> Counter/1, Delay1/1
  Constant/1 -> Relational/2
  Relational/1 -> reg_bs0/2, reg_bs1/2
  reg_bs0/1 -> reghold_bs0/1
  reg_bs1/1 -> reghold_bs1/1
  Delay1/1 -> sync_out/1, monitor_2x16/1(sync)
  reghold_bs0/1 -> bs0/1, monitor_2x16/2(bs0)
  reghold_bs1/1 -> bs1/1, monitor_2x16/3(bs1)
  Counter/1 -> Slice32/1, Slice33/1
  Slice32/1 -> Relational/1
  Constant1/1 -> Relational1/2
  Slice33/1 -> Relational1/1
  Relational1/1 -> Delay2/1
  Delay2/1 -> reghold_bs0/2, reghold_bs1/2

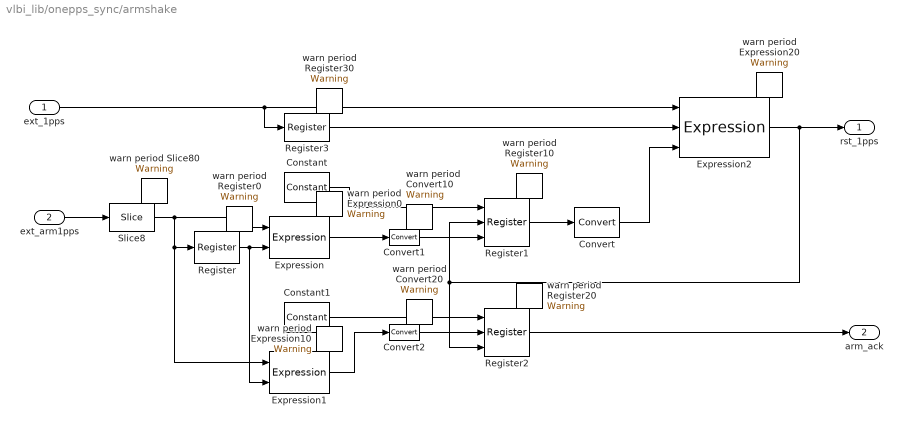
== system vlbi_lib/onepps_sync/armshake ==
  ext_1pps : Inport  OutDataType=sfix(16)  OutScaling=2^0
  ext_arm1pps : Inport  Port=2  OutDataType=sfix(16)  OutScaling=2^0
  Constant : xbsIndex_r4/Constant  arith_type=Unsigned  const=1  n_bits=1  bin_pt=0  explicit_period=on  period=1  equ=P=C  opselect=C  inp2=PCIN>>17  opr=+  inp1=P  carry=CIN  dbl_ovrd=off  block_type=constant
      settings: block_version=11.3
  Constant1 : xbsIndex_r4/Constant  arith_type=Unsigned  const=1  n_bits=1  bin_pt=0  explicit_period=on  period=1  equ=P=C  opselect=C  inp2=PCIN>>17  opr=+  inp1=P  carry=CIN  dbl_ovrd=off  block_type=constant
      settings: block_version=11.3
  Convert : xbsIndex_r4/Convert  arith_type=Boolean  n_bits=8  bin_pt=6  quantization=Truncate  overflow=Wrap  latency=0  dbl_ovrd=off  pipeline=off  block_type=convert
      settings: xl_area=[0, 0, 0, 0, 0, 0, 0]  block_version=11.3
  Convert1 : xbsIndex_r4/Convert  arith_type=Boolean  n_bits=8  bin_pt=6  quantization=Truncate  overflow=Wrap  latency=0  dbl_ovrd=off  pipeline=off  block_type=convert
      settings: xl_area=[0, 0, 0, 0, 0, 0, 0]  block_version=11.3
  Convert2 : xbsIndex_r4/Convert  arith_type=Boolean  n_bits=8  bin_pt=6  quantization=Truncate  overflow=Wrap  latency=0  dbl_ovrd=off  pipeline=off  block_type=convert
      settings: xl_area=[0, 0, 0, 0, 0, 0, 0]  block_version=11.3
  Expression : xbsIndex_r4/Expression  expression=a & ~b  align_bp=on  en=off  latency=0  precision=Full  arith_type=Unsigned  n_bits=8  bin_pt=2  dbl_ovrd=off  block_type=expr
      settings: xl_area=[0, 0, 0, 0, 0, 0, 0]  block_version=11.3
  Expression1 : xbsIndex_r4/Expression  expression=~a & b  align_bp=on  en=off  latency=0  precision=Full  arith_type=Unsigned  n_bits=8  bin_pt=2  dbl_ovrd=off  block_type=expr
      settings: xl_area=[0, 0, 0, 0, 0, 0, 0]  block_version=11.3
  Expression2 : xbsIndex_r4/Expression  expression=(a & ~b) & c  align_bp=on  en=off  latency=1  precision=Full  arith_type=Unsigned  n_bits=8  bin_pt=2  dbl_ovrd=off  block_type=expr
      settings: xl_area=[0, 0, 0, 0, 0, 0, 0]  block_version=11.3
  Register : xbsIndex_r4/Register  init=0  rst=off  en=off  dbl_ovrd=off  block_type=register
      settings: xl_area=[0, 0, 0, 0, 0, 0, 0]  block_version=11.3
  Register1 : xbsIndex_r4/Register  init=0  rst=on  en=on  dbl_ovrd=off  block_type=register
      settings: xl_area=[0, 0, 0, 0, 0, 0, 0]  block_version=11.3
  Register2 : xbsIndex_r4/Register  init=0  rst=on  en=on  dbl_ovrd=off  block_type=register
      settings: xl_area=[0, 0, 0, 0, 0, 0, 0]  block_version=11.3
  Register3 : xbsIndex_r4/Register  init=0  rst=off  en=off  dbl_ovrd=off  block_type=register
      settings: xl_area=[0, 0, 0, 0, 0, 0, 0]  block_version=11.3
  Slice8 : xbsIndex_r4/Slice  nbits=1  boolean_output=off  mode=Lower Bit Location + Width  bit1=0  base1=MSB of Input  bit0=0  base0=LSB of Input  dbl_ovrd=off  block_type=slice
      settings: block_version=11.3
  warn period Convert10 : xbsReplacements_r4/Warning  SystemSampleTime=-1  period=1
  warn period Convert20 : xbsReplacements_r4/Warning  SystemSampleTime=-1  period=1
  warn period Expression0 : xbsReplacements_r4/Warning  SystemSampleTime=-1  period=1
  warn period Expression10 : xbsReplacements_r4/Warning  SystemSampleTime=-1  period=1
  warn period Expression20 : xbsReplacements_r4/Warning  SystemSampleTime=-1  period=1
  warn period Register{0,10,20,30} (4 alike) : xbsReplacements_r4/Warning  SystemSampleTime=-1  period=1
  warn period Slice80 : xbsReplacements_r4/Warning  SystemSampleTime=-1  period=1
  rst_1pps : Outport  OutDataType=sfix(16)  OutScaling=2^0
  arm_ack : Outport  Port=2  OutDataType=sfix(16)  OutScaling=2^0
  wires:
  Convert2/1 -> Register2/2
  Convert1/1 -> Register1/3
  Register2/1 -> arm_ack/1
  Expression1/1 -> Convert2/1
  Constant1/1 -> Register2/1
  Expression/1 -> Convert1/1
  Constant/1 -> Register1/1
  ext_arm1pps/1 -> Slice8/1
  Expression2/1 -> Register2/3, Register1/2, rst_1pps/1
  ext_1pps/1 -> Register3/1, Expression2/1
  Register1/1 -> Convert/1
  Slice8/1 -> Expression1/1, Register/1, Expression/1
  Register3/1 -> Expression2/2
  Convert/1 -> Expression2/3
  Register/1 -> Expression1/2, Expression/2

== system vlbi_lib/onepps_sync/int_1pps_gen ==
  rst : Inport  OutDataType=sfix(16)  OutScaling=2^0
  1pps_gen : Subsystem
  Simulation Multiplexer : xbsIndex_r4/Simulation Multiplexer  sim_sel=2  hw_sel=1  block_type=simmux
      settings: infoedit="Distinguish input subsystems as \"simulation only\" and \"generation only\".  The input specified For Simulation will be used during Simulink simulation.  The input specified For Generation will be used during code generation.  This block will typically be used on the output of a HW Co-Simulation, Black Box, or ModelSim subsystem.<br><br>Hardware Notes: This block costs nothing."  block_version=11.3
  sim1pps_gen : Subsystem
  1pps : Outport  OutDataType=sfix(16)  OutScaling=2^0
  wires:
  1pps_gen/1(1pps) -> Simulation Multiplexer/1
  sim1pps_gen/1(1pps_sim) -> Simulation Multiplexer/2
  rst/1 -> 1pps_gen/1(rst), sim1pps_gen/1(rst)
  Simulation Multiplexer/1 -> 1pps/1

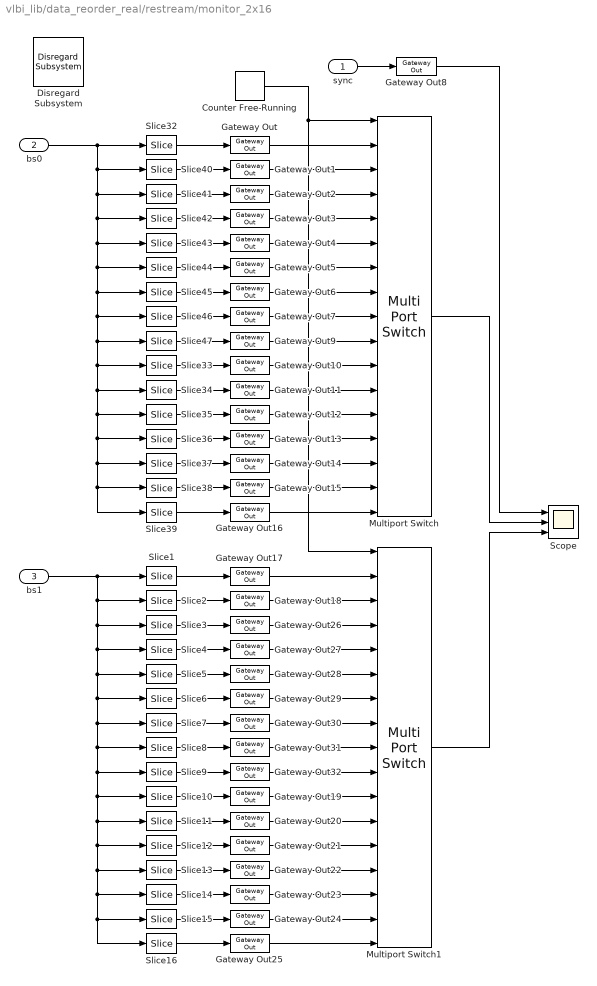
== system vlbi_lib/data_reorder_real/restream/monitor_2x16 ==
  sync : Inport  OutDataType=sfix(16)  OutScaling=2^0
  bs0 : Inport  Port=2  OutDataType=sfix(16)  OutScaling=2^0
  bs1 : Inport  Port=3  OutDataType=sfix(16)  OutScaling=2^0
  Counter Free-Running : simulink/Sources/Counter Free-Running  SystemSampleTime=-1  NumBits=4  tsamp=1/16
  Disregard Subsystem : xbsIndex_r4/Disregard Subsystem  Tag=discardX  block_type=disregard
      settings: block_version=11.3
  Gateway Out{,1..32} (33 alike) : xbsIndex_r4/Gateway Out  hdl_port=off  timing_constraint=None  locs_specified=off  LOCs={}  block_type=gatewayout
      settings: infoedit="Gateway out block.  Converts Xilinx fixed point inputs into ouputs of type Simulink integer, double, or fixed point.<br><br>Hardware notes:  In hardware these blocks become top level output ports or are discarded, depending on how they are configured."  xl_area=[0, 0, 0, 0, 0, 0, 0]  block_version=11.3
  Multiport Switch : MultiPortSwitch  Inputs=16  zeroidx=on  SampleTime=1/16
  Multiport Switch1 : MultiPortSwitch  Inputs=16  zeroidx=on  SampleTime=1/16
  Scope : Scope  NumInputPorts=3
      settings: YMin=-5~-5~-5  YMax=5~5~5
  Slice1 : xbsIndex_r4/Slice  nbits=sample_width  boolean_output=off  mode=Upper Bit Location + Width  bit1=sample_width * 0  base1=MSB of Input  bit0=0  base0=LSB of Input  dbl_ovrd=off  block_type=slice
      settings: block_version=11.3
  Slice10 : xbsIndex_r4/Slice  nbits=sample_width  boolean_output=off  mode=Upper Bit Location + Width  bit1=sample_width * -9  base1=MSB of Input  bit0=0  base0=LSB of Input  dbl_ovrd=off  block_type=slice
      settings: block_version=11.3
  Slice11 : xbsIndex_r4/Slice  nbits=sample_width  boolean_output=off  mode=Upper Bit Location + Width  bit1=sample_width * -10  base1=MSB of Input  bit0=0  base0=LSB of Input  dbl_ovrd=off  block_type=slice
      settings: block_version=11.3
  Slice12 : xbsIndex_r4/Slice  nbits=sample_width  boolean_output=off  mode=Upper Bit Location + Width  bit1=sample_width * -11  base1=MSB of Input  bit0=0  base0=LSB of Input  dbl_ovrd=off  block_type=slice
      settings: block_version=11.3
  Slice13 : xbsIndex_r4/Slice  nbits=sample_width  boolean_output=off  mode=Upper Bit Location + Width  bit1=sample_width * -12  base1=MSB of Input  bit0=0  base0=LSB of Input  dbl_ovrd=off  block_type=slice
      settings: block_version=11.3
  Slice14 : xbsIndex_r4/Slice  nbits=sample_width  boolean_output=off  mode=Upper Bit Location + Width  bit1=sample_width * -13  base1=MSB of Input  bit0=0  base0=LSB of Input  dbl_ovrd=off  block_type=slice
      settings: block_version=11.3
  Slice15 : xbsIndex_r4/Slice  nbits=sample_width  boolean_output=off  mode=Upper Bit Location + Width  bit1=sample_width * -14  base1=MSB of Input  bit0=0  base0=LSB of Input  dbl_ovrd=off  block_type=slice
      settings: block_version=11.3
  Slice16 : xbsIndex_r4/Slice  nbits=sample_width  boolean_output=off  mode=Upper Bit Location + Width  bit1=sample_width * -15  base1=MSB of Input  bit0=0  base0=LSB of Input  dbl_ovrd=off  block_type=slice
      settings: block_version=11.3
  Slice2 : xbsIndex_r4/Slice  nbits=sample_width  boolean_output=off  mode=Upper Bit Location + Width  bit1=sample_width * -1  base1=MSB of Input  bit0=0  base0=LSB of Input  dbl_ovrd=off  block_type=slice
      settings: block_version=11.3
  Slice3 : xbsIndex_r4/Slice  nbits=sample_width  boolean_output=off  mode=Upper Bit Location + Width  bit1=sample_width * -2  base1=MSB of Input  bit0=0  base0=LSB of Input  dbl_ovrd=off  block_type=slice
      settings: block_version=11.3
  Slice32 : xbsIndex_r4/Slice  nbits=sample_width  boolean_output=off  mode=Upper Bit Location + Width  bit1=sample_width * 0  base1=MSB of Input  bit0=0  base0=LSB of Input  dbl_ovrd=off  block_type=slice
      settings: block_version=11.3
  Slice33 : xbsIndex_r4/Slice  nbits=sample_width  boolean_output=off  mode=Upper Bit Location + Width  bit1=sample_width * -9  base1=MSB of Input  bit0=0  base0=LSB of Input  dbl_ovrd=off  block_type=slice
      settings: block_version=11.3
  Slice34 : xbsIndex_r4/Slice  nbits=sample_width  boolean_output=off  mode=Upper Bit Location + Width  bit1=sample_width * -10  base1=MSB of Input  bit0=0  base0=LSB of Input  dbl_ovrd=off  block_type=slice
      settings: block_version=11.3
  Slice35 : xbsIndex_r4/Slice  nbits=sample_width  boolean_output=off  mode=Upper Bit Location + Width  bit1=sample_width * -11  base1=MSB of Input  bit0=0  base0=LSB of Input  dbl_ovrd=off  block_type=slice
      settings: block_version=11.3
  Slice36 : xbsIndex_r4/Slice  nbits=sample_width  boolean_output=off  mode=Upper Bit Location + Width  bit1=sample_width * -12  base1=MSB of Input  bit0=0  base0=LSB of Input  dbl_ovrd=off  block_type=slice
      settings: block_version=11.3
  Slice37 : xbsIndex_r4/Slice  nbits=sample_width  boolean_output=off  mode=Upper Bit Location + Width  bit1=sample_width * -13  base1=MSB of Input  bit0=0  base0=LSB of Input  dbl_ovrd=off  block_type=slice
      settings: block_version=11.3
  Slice38 : xbsIndex_r4/Slice  nbits=sample_width  boolean_output=off  mode=Upper Bit Location + Width  bit1=sample_width * -14  base1=MSB of Input  bit0=0  base0=LSB of Input  dbl_ovrd=off  block_type=slice
      settings: block_version=11.3
  Slice39 : xbsIndex_r4/Slice  nbits=sample_width  boolean_output=off  mode=Upper Bit Location + Width  bit1=sample_width * -15  base1=MSB of Input  bit0=0  base0=LSB of Input  dbl_ovrd=off  block_type=slice
      settings: block_version=11.3
  Slice4 : xbsIndex_r4/Slice  nbits=sample_width  boolean_output=off  mode=Upper Bit Location + Width  bit1=sample_width * -3  base1=MSB of Input  bit0=0  base0=LSB of Input  dbl_ovrd=off  block_type=slice
      settings: block_version=11.3
  Slice40 : xbsIndex_r4/Slice  nbits=sample_width  boolean_output=off  mode=Upper Bit Location + Width  bit1=sample_width * -1  base1=MSB of Input  bit0=0  base0=LSB of Input  dbl_ovrd=off  block_type=slice
      settings: block_version=11.3
  Slice41 : xbsIndex_r4/Slice  nbits=sample_width  boolean_output=off  mode=Upper Bit Location + Width  bit1=sample_width * -2  base1=MSB of Input  bit0=0  base0=LSB of Input  dbl_ovrd=off  block_type=slice
      settings: block_version=11.3
  Slice42 : xbsIndex_r4/Slice  nbits=sample_width  boolean_output=off  mode=Upper Bit Location + Width  bit1=sample_width * -3  base1=MSB of Input  bit0=0  base0=LSB of Input  dbl_ovrd=off  block_type=slice
      settings: block_version=11.3
  Slice43 : xbsIndex_r4/Slice  nbits=sample_width  boolean_output=off  mode=Upper Bit Location + Width  bit1=sample_width * -4  base1=MSB of Input  bit0=0  base0=LSB of Input  dbl_ovrd=off  block_type=slice
      settings: block_version=11.3
  Slice44 : xbsIndex_r4/Slice  nbits=sample_width  boolean_output=off  mode=Upper Bit Location + Width  bit1=sample_width * -5  base1=MSB of Input  bit0=0  base0=LSB of Input  dbl_ovrd=off  block_type=slice
      settings: block_version=11.3
  Slice45 : xbsIndex_r4/Slice  nbits=sample_width  boolean_output=off  mode=Upper Bit Location + Width  bit1=sample_width * -6  base1=MSB of Input  bit0=0  base0=LSB of Input  dbl_ovrd=off  block_type=slice
      settings: block_version=11.3
  Slice46 : xbsIndex_r4/Slice  nbits=sample_width  boolean_output=off  mode=Upper Bit Location + Width  bit1=sample_width * -7  base1=MSB of Input  bit0=0  base0=LSB of Input  dbl_ovrd=off  block_type=slice
      settings: block_version=11.3
  Slice47 : xbsIndex_r4/Slice  nbits=sample_width  boolean_output=off  mode=Upper Bit Location + Width  bit1=sample_width * -8  base1=MSB of Input  bit0=0  base0=LSB of Input  dbl_ovrd=off  block_type=slice
      settings: block_version=11.3
  Slice5 : xbsIndex_r4/Slice  nbits=sample_width  boolean_output=off  mode=Upper Bit Location + Width  bit1=sample_width * -4  base1=MSB of Input  bit0=0  base0=LSB of Input  dbl_ovrd=off  block_type=slice
      settings: block_version=11.3
  Slice6 : xbsIndex_r4/Slice  nbits=sample_width  boolean_output=off  mode=Upper Bit Location + Width  bit1=sample_width * -5  base1=MSB of Input  bit0=0  base0=LSB of Input  dbl_ovrd=off  block_type=slice
      settings: block_version=11.3
  Slice7 : xbsIndex_r4/Slice  nbits=sample_width  boolean_output=off  mode=Upper Bit Location + Width  bit1=sample_width * -6  base1=MSB of Input  bit0=0  base0=LSB of Input  dbl_ovrd=off  block_type=slice
      settings: block_version=11.3
  Slice8 : xbsIndex_r4/Slice  nbits=sample_width  boolean_output=off  mode=Upper Bit Location + Width  bit1=sample_width * -7  base1=MSB of Input  bit0=0  base0=LSB of Input  dbl_ovrd=off  block_type=slice
      settings: block_version=11.3
  Slice9 : xbsIndex_r4/Slice  nbits=sample_width  boolean_output=off  mode=Upper Bit Location + Width  bit1=sample_width * -8  base1=MSB of Input  bit0=0  base0=LSB of Input  dbl_ovrd=off  block_type=slice
      settings: block_version=11.3
  wires:
  Counter Free-Running/1 -> Multiport Switch/1, Multiport Switch1/1
  Slice46/1 -> Gateway Out7/1
  Slice45/1 -> Gateway Out6/1
  Slice44/1 -> Gateway Out5/1
  Slice43/1 -> Gateway Out4/1
  Slice42/1 -> Gateway Out3/1
  Slice41/1 -> Gateway Out2/1
  Slice40/1 -> Gateway Out1/1
  Slice32/1 -> Gateway Out/1
  bs0/1 -> Slice38/1, Slice39/1, Slice37/1, Slice36/1, Slice35/1, Slice34/1, Slice33/1, Slice47/1, Slice46/1, Slice45/1, Slice44/1, Slice43/1, Slice42/1, Slice41/1, Slice40/1, Slice32/1
  Slice39/1 -> Gateway Out16/1
  Slice38/1 -> Gateway Out15/1
  Slice37/1 -> Gateway Out14/1
  Slice36/1 -> Gateway Out13/1
  Slice35/1 -> Gateway Out12/1
  Slice34/1 -> Gateway Out11/1
  Slice33/1 -> Gateway Out10/1
  Slice47/1 -> Gateway Out9/1
  Slice8/1 -> Gateway Out31/1
  Slice7/1 -> Gateway Out30/1
  Slice6/1 -> Gateway Out29/1
  Slice5/1 -> Gateway Out28/1
  Slice4/1 -> Gateway Out27/1
  Slice3/1 -> Gateway Out26/1
  Slice2/1 -> Gateway Out18/1
  Slice1/1 -> Gateway Out17/1
  Slice16/1 -> Gateway Out25/1
  Slice15/1 -> Gateway Out24/1
  Slice14/1 -> Gateway Out23/1
  Slice13/1 -> Gateway Out22/1
  Slice12/1 -> Gateway Out21/1
  Slice11/1 -> Gateway Out20/1
  Slice10/1 -> Gateway Out19/1
  Slice9/1 -> Gateway Out32/1
  Gateway Out/1 -> Multiport Switch/2
  Gateway Out1/1 -> Multiport Switch/3
  Gateway Out2/1 -> Multiport Switch/4
  Gateway Out3/1 -> Multiport Switch/5
  Gateway Out4/1 -> Multiport Switch/6
  Gateway Out5/1 -> Multiport Switch/7
  Gateway Out6/1 -> Multiport Switch/8
  Gateway Out7/1 -> Multiport Switch/9
  Gateway Out9/1 -> Multiport Switch/10
  Gateway Out10/1 -> Multiport Switch/11
  Gateway Out11/1 -> Multiport Switch/12
  Gateway Out12/1 -> Multiport Switch/13
  Gateway Out13/1 -> Multiport Switch/14
  Gateway Out14/1 -> Multiport Switch/15
  Gateway Out15/1 -> Multiport Switch/16
  Gateway Out16/1 -> Multiport Switch/17
  Gateway Out17/1 -> Multiport Switch1/2
  Gateway Out18/1 -> Multiport Switch1/3
  Gateway Out26/1 -> Multiport Switch1/4
  Gateway Out27/1 -> Multiport Switch1/5
  Gateway Out28/1 -> Multiport Switch1/6
  Gateway Out29/1 -> Multiport Switch1/7
  Gateway Out30/1 -> Multiport Switch1/8
  Gateway Out31/1 -> Multiport Switch1/9
  Gateway Out32/1 -> Multiport Switch1/10
  Gateway Out19/1 -> Multiport Switch1/11
  Gateway Out20/1 -> Multiport Switch1/12
  Gateway Out21/1 -> Multiport Switch1/13
  Gateway Out22/1 -> Multiport Switch1/14
  Gateway Out23/1 -> Multiport Switch1/15
  Gateway Out24/1 -> Multiport Switch1/16
  Gateway Out25/1 -> Multiport Switch1/17
  sync/1 -> Gateway Out8/1
  Gateway Out8/1 -> Scope/1
  Multiport Switch/1 -> Scope/2
  Multiport Switch1/1 -> Scope/3
  bs1/1 -> Slice1/1, Slice2/1, Slice3/1, Slice4/1, Slice5/1, Slice6/1, Slice7/1, Slice8/1, Slice9/1, Slice10/1, Slice11/1, Slice12/1, Slice13/1, Slice14/1, Slice15/1, Slice16/1

== system vlbi_lib/onepps_sync/int_1pps_gen/1pps_gen ==
  rst : Inport  OutDataType=sfix(16)  OutScaling=2^0
  Constant : xbsIndex_r4/Constant  arith_type=Unsigned  const=0  n_bits=32  bin_pt=0  explicit_period=on  period=1  equ=P=C  opselect=C  inp2=PCIN>>17  opr=+  inp1=P  carry=CIN  dbl_ovrd=off  block_type=constant
      settings: block_version=11.3
  Counter : xbsIndex_r4/Counter  cnt_type=Count Limited  cnt_to=256000000-1  operation=Up  start_count=0  cnt_by_val=1  arith_type=Unsigned  n_bits=32  bin_pt=0  load_pin=off  rst=on  en=off  explicit_period=off  period=1  dbl_ovrd=off  use_behavioral_HDL=off  implementation=Fabric  use_rpm=on  block_type=counter
      settings: xl_area=[0, 0, 0, 0, 0, 0, 0]  block_version=11.3
  Relational : xbsIndex_r4/Relational  mode=a=b  en=off  latency=1  dbl_ovrd=off  block_type=relational
      settings: xl_area=[0, 0, 0, 0, 0, 0, 0]  block_version=11.3
  warn period Relational0 : xbsReplacements_r4/Warning  SystemSampleTime=-1  period=1
  1pps : Outport  OutDataType=sfix(16)  OutScaling=2^0
  wires:
  Constant/1 -> Relational/2
  Counter/1 -> Relational/1
  rst/1 -> Counter/1
  Relational/1 -> 1pps/1

== system vlbi_lib/onepps_sync/int_1pps_gen/sim1pps_gen ==
  rst : Inport  OutDataType=sfix(16)  OutScaling=2^0
  Constant : xbsIndex_r4/Constant  arith_type=Unsigned  const=0  n_bits=28  bin_pt=0  explicit_period=on  period=1  equ=P=C  opselect=C  inp2=PCIN>>17  opr=+  inp1=P  carry=CIN  dbl_ovrd=off  block_type=constant
      settings: block_version=11.3
  Counter : xbsIndex_r4/Counter  cnt_type=Count Limited  cnt_to=2560-1  operation=Up  start_count=0  cnt_by_val=1  arith_type=Unsigned  n_bits=28  bin_pt=0  load_pin=off  rst=on  en=off  explicit_period=off  period=1  dbl_ovrd=off  use_behavioral_HDL=off  implementation=Fabric  use_rpm=on  block_type=counter
      settings: xl_area=[0, 0, 0, 0, 0, 0, 0]  block_version=11.3
  Disregard Subsystem : xbsIndex_r4/Disregard Subsystem  Tag=discardX  block_type=disregard
      settings: block_version=11.3
  Relational : xbsIndex_r4/Relational  mode=a=b  en=off  latency=1  dbl_ovrd=off  block_type=relational
      settings: xl_area=[0, 0, 0, 0, 0, 0, 0]  block_version=11.3
  1pps_sim : Outport  OutDataType=sfix(16)  OutScaling=2^0
  wires:
  Relational/1 -> 1pps_sim/1
  rst/1 -> Counter/1
  Counter/1 -> Relational/1
  Constant/1 -> Relational/2
